simulink model "EKF_MODEL_needfix"  (R2023b)
settings: Solver=ode23tb  StartTime=0.0  StopTime=30  FixedStep=.001  RelTol=2e-1  EnableMultiTasking=on
StartFcn:
  | %tic
StopFcn:
  | %toc
model workspace (MAT data in the model file):
  DLCXref = [0 6.1 6.2 18 33 33.5 45 50 60]
  DLCXrefStanley = [0 1.2 2.4 3.6 4.8 6 7.2 8.4 9.44987166868 10.0991210544 10.1 10.1008789456 ... (38 elements, 1x38)]
  DLCYref = [0 0 -5 -3.875 -3.5 1 0 0 0]
  DLCYrefStanley = [0.1375 0.1375 0.1375 0.1375 0.1375 0.1375 0.1375 0.1375 -0.203439148031 -1.09615705337 -2.2 -3.30384294663 ... (38 elements, 1x38)]
  Downshift_Speeds = [9.5625 12.9375 16.3125 19.6875 23.0625 26.4375 29.8125 33.1875 36.5625 39.9375 43.3125 46.6875 ... (28 elements, 4x7)]
  EngRevLim = 7000
  Pedal_Positions = [0.1 0.4 0.5 0.9]
  Ts = 0.01
  Upshift_Speeds = [12.9375 16.3125 19.6875 33 26.4375 29.8125 33.1875 52.5 39.9375 43.3125 46.6875 77.25 ... (28 elements, 4x7)]
  VEH : object (value not decoded)
  a = 1.515
  b = 1.504
  for_ekf : mamfis (value not decoded)
  rayDirections = [0 0 0 0 0 0 0 0 0 0 0 0 ... (363 elements, 121x3)]
  rayLengths = [20 20 20 20 20 20 20 20 20 20 20 20 ... (121 elements, 121x1)]
  rayOrigins = [0.5 0.4 0.3 0.2 0.1 0 -0.1 -0.2 -0.3 -0.4 -0.5 0.5 ... (363 elements, 121x3)]
  theta = 1
  wf = 0.75
  wr = 1.25
symbols that are objects in the model workspace (value not decoded): VEH
undefined symbols (not defined in the file): DiscIntNeverNeededParam
libraries: simulink x14, autolibutils x7, slpidlib x2, vehdynlibdriver x2, vehdynlibviscommon x2, sim3dgroundtruthsensorlib x2, autolibtranscontrolscommon x1, autolibshared x1, sharedtransform x1, sharedTrackingLibrary x1, vehdynlibscenariocommon x1, vehdynlibsens x1
(part 4 of 4)

== system EKF_MODEL_needfix/Visualization/3D Engine/3D Engine/Part Translation Concatenation ==
  BodyX : Inport
  BodyY : Inport  Port=2
  BodyZ : Inport  Port=3
  WheelFrontLeftX : Inport  Port=4
  WheelFrontRightX : Inport  Port=5
  WheelRearLeftX : Inport  Port=6
  WheelRearRightX : Inport  Port=7
  WheelFrontLeftY : Inport  Port=8
  WheelFrontRightY : Inport  Port=9
  WheelRearLeftY : Inport  Port=10
  WheelRearRightY : Inport  Port=11
  WheelFrontLeftZ : Inport  Port=12
  WheelFrontRightZ : Inport  Port=13
  WheelRearLeftZ : Inport  Port=14
  WheelRearRightZ : Inport  Port=15
  AllParts : Concatenate  NumInputs=5  Mode=Multidimensional array
  Body : Concatenate  NumInputs=3  Mode=Multidimensional array  ConcatenateDimension=2
  WheelFrontLeft : Concatenate  NumInputs=3  Mode=Multidimensional array  ConcatenateDimension=2
  WheelFrontRight : Concatenate  NumInputs=3  Mode=Multidimensional array  ConcatenateDimension=2
  WheelRearLeft : Concatenate  NumInputs=3  Mode=Multidimensional array  ConcatenateDimension=2
  WheelRearRight : Concatenate  NumInputs=3  Mode=Multidimensional array  ConcatenateDimension=2
  ConcatOut : Outport  VectorParamsAs1DForOutWhenUnconnected=off
  wires:
  BodyX/1 -> Body/1
  BodyZ/1 -> Body/3
  WheelFrontLeftX/1 -> WheelFrontLeft/1
  WheelFrontLeftZ/1 -> WheelFrontLeft/3
  WheelFrontLeftY/1 -> WheelFrontLeft/2
  BodyY/1 -> Body/2
  WheelFrontLeft/1 -> AllParts/2
  WheelRearRightX/1 -> WheelRearRight/1
  Body/1 -> AllParts/1
  WheelRearLeft/1 -> AllParts/4
  WheelFrontRight/1 -> AllParts/3
  WheelRearRightZ/1 -> WheelRearRight/3
  WheelFrontRightY/1 -> WheelFrontRight/2
  WheelFrontRightX/1 -> WheelFrontRight/1
  WheelRearRightY/1 -> WheelRearRight/2
  WheelRearLeftZ/1 -> WheelRearLeft/3
  AllParts/1 -> ConcatOut/1
  WheelRearLeftY/1 -> WheelRearLeft/2
  WheelRearRight/1 -> AllParts/5
  WheelRearLeftX/1 -> WheelRearLeft/1
  WheelFrontRightZ/1 -> WheelFrontRight/3

== system EKF_MODEL_needfix/Visualization/3D Engine/3D Engine/Scale ==
  Constant{1..12,17,32..33} (15 alike) : Constant  OutDataTypeStr=single
  PartConcatenation : Subsystem
  ScaleOut : Outport  VectorParamsAs1DForOutWhenUnconnected=off
  wires:
  Constant10/1 -> PartConcatenation/15(WheelRearRightZ)
  Constant9/1 -> PartConcatenation/14(WheelRearRightY)
  Constant11/1 -> PartConcatenation/13(WheelRearRightX)
  Constant7/1 -> PartConcatenation/12(WheelRearLeftZ)
  Constant6/1 -> PartConcatenation/11(WheelRearLeftY)
  Constant8/1 -> PartConcatenation/10(WheelRearLeftX)
  Constant4/1 -> PartConcatenation/9(WheelFrontRightZ)
  Constant3/1 -> PartConcatenation/8(WheelFrontRightY)
  Constant5/1 -> PartConcatenation/7(WheelFrontRightX)
  Constant2/1 -> PartConcatenation/6(WheelFrontLeftZ)
  Constant1/1 -> PartConcatenation/5(WheelFrontLeftY)
  Constant33/1 -> PartConcatenation/4(WheelFrontLeftX)
  Constant32/1 -> PartConcatenation/3(BodyZ)
  Constant17/1 -> PartConcatenation/2(BodyY)
  Constant12/1 -> PartConcatenation/1(BodyX)
  PartConcatenation/1(ConcatOut) -> ScaleOut/1

== system EKF_MODEL_needfix/Controllers/Brake Pressure Control/Five-State ABS and TCS/ABSCtrlForEach/For Each Subsystem ==
  e1 : Inport  Partition=on  PartitionDimension=1  PartitionWidth=1  PartitionOffset=0
  e2 : Inport  Port=2  Partition=on  PartitionDimension=1  PartitionWidth=1  PartitionOffset=0
  Pref : Inport  Port=3  Partition=on  PartitionDimension=1  PartitionWidth=1  PartitionOffset=0
  VehSpd : Inport  Port=4
  ABSForEachWheel : Stateflow chart  InitFcn=[~]=vehdynicon('vehdynblk',gcb);  TreatAsAtomicUnit=on
  For Each : ForEach  DisableCoverage=on
  Saturation2 : Saturate  UpperLimit=1  LowerLimit=0  ZeroCross=off
  Pb : Outport  ConcatenationDimension=1
  Flag : Outport  Port=2  ConcatenationDimension=1
  wires:
  e1/1 -> ABSForEachWheel/1(e1)
  e2/1 -> ABSForEachWheel/2(e2)
  VehSpd/1 -> ABSForEachWheel/4(VehSpd)
  Saturation2/1 -> Pb/1  "BrkPrsCmdCtrl"
  ABSForEachWheel/2(Flag) -> Flag/1
  ABSForEachWheel/1(PbOutput) -> Saturation2/1
  Pref/1 -> ABSForEachWheel/3(Pref)

== system EKF_MODEL_needfix/Controllers/Brake Pressure Control/Five-State ABS and TCS/TCSCtrlForEach/For Each Subsystem ==
  e1 : Inport  Partition=on  PartitionDimension=1  PartitionWidth=1  PartitionOffset=0
  Enb : Inport  Port=2
  e2 : Inport  Port=3  Partition=on  PartitionDimension=1  PartitionWidth=1  PartitionOffset=0
  AccelFdbk : Inport  Port=4  Partition=on  PartitionDimension=1  PartitionWidth=1  PartitionOffset=0
  PbFdbk : Inport  Port=5  Partition=on  PartitionDimension=1  PartitionWidth=1  PartitionOffset=0
  ABSForEachWheel : Stateflow chart  InitFcn=[~]=vehdynicon('vehdynblk',gcb);  TreatAsAtomicUnit=on
  Discrete-Time Integrator1 : DiscreteIntegrator  IntegratorMethod=Integration: Trapezoidal  ExternalReset=rising  SampleTime=-1  LimitOutput=on  UpperSaturationLimit=1  LowerSaturationLimit=0  ICPrevOutput=DiscIntNeverNeededParam  ICPrevScaledInput=DiscIntNeverNeededParam
  For Each : ForEach  DisableCoverage=on
  IsNegative : simulink/Logic and Bit Operations/Compare To Zero  relop===  OutDataTypeStr=boolean  ZeroCross=off
  Pb : Outport  ConcatenationDimension=1
  Flag : Outport  Port=2  ConcatenationDimension=1
  wires:
  e1/1 -> ABSForEachWheel/1(e1)
  e2/1 -> ABSForEachWheel/2(e2)
  Discrete-Time Integrator1/1 -> Pb/1  "BrkPrsCmdCtrl"
  ABSForEachWheel/2(Flag) -> IsNegative/1, Flag/1
  ABSForEachWheel/1(PbOutput) -> Discrete-Time Integrator1/1
  AccelFdbk/1 -> ABSForEachWheel/3(AccelFdbk)
  Enb/1 -> ABSForEachWheel/4(Enb)
  PbFdbk/1 -> ABSForEachWheel/5(Pb)
  IsNegative/1 -> Discrete-Time Integrator1/2

== system EKF_MODEL_needfix/Controllers/Brake Pressure Control/Five-State ABS and TCS/Wheel Accel and Slip Estimator/Kappa ==
  xdot : Inport
  Omega : Inport  Port=2  PortDimensions=1  Partition=on  PartitionDimension=1  PartitionWidth=1  PartitionOffset=0
  For Each : ForEach  DisableCoverage=on
  MATLAB Function : MATLAB Function  TreatAsAtomicUnit=on
  KappaEst : Outport  ConcatenationDimension=1
  wires:
  MATLAB Function/1(KappaEst) -> KappaEst/1
  xdot/1 -> MATLAB Function/2(xdot)
  Omega/1 -> MATLAB Function/1(Omega)

== system EKF_MODEL_needfix/Controllers/Brake Pressure Control/Five-State ABS and TCS/Wheel Accel and Slip Estimator/Wheel Accel ==
  Omega : Inport  PortDimensions=1  Partition=on  PartitionDimension=1  PartitionWidth=1  PartitionOffset=0
  For Each : ForEach  DisableCoverage=on
  SG Diff : autolibutils/SG Diff  N=2  F=500  div0Tol=.001  aMode=2
  Terminator : Terminator
  WhlAccel : Outport  ConcatenationDimension=1
  wires:
  Omega/1 -> SG Diff/1
  SG Diff/1 -> Terminator/1
  SG Diff/2 -> WhlAccel/1

== system EKF_MODEL_needfix/Controllers/Transmission Controller/Transmission Controller/TCM/Neutral Select ==
  AccCmd : Inport
  EngSpd : Inport  Port=2
  Constant : Constant  Value=1200
  Constant1 : Constant  Value=1e-2
  Constant2 : Constant  Value=500
  Logical Operator : Logic  AllPortsSameDT=off  OutDataTypeStr=boolean
  Logical Operator1 : Logic  Operator=OR  AllPortsSameDT=off  OutDataTypeStr=boolean
  Relational Operator : RelationalOperator  Operator=<=  OutDataTypeStr=boolean  ZeroCross=off  RndMeth=Simplest  InputSameDT=off
  Relational Operator1 : RelationalOperator  Operator=<=  OutDataTypeStr=boolean  ZeroCross=off  RndMeth=Simplest  InputSameDT=off
  Relational Operator2 : RelationalOperator  Operator=<=  OutDataTypeStr=boolean  ZeroCross=off  RndMeth=Simplest  InputSameDT=off
  Neutral Select : Outport  VectorParamsAs1DForOutWhenUnconnected=off
  wires:
  EngSpd/1 -> Relational Operator/1, Relational Operator2/1
  Relational Operator1/1 -> Logical Operator/1
  AccCmd/1 -> Relational Operator1/1
  Constant1/1 -> Relational Operator1/2
  Logical Operator1/1 -> Neutral Select/1
  Constant/1 -> Relational Operator/2
  Relational Operator/1 -> Logical Operator/2
  Logical Operator/1 -> Logical Operator1/1
  Constant2/1 -> Relational Operator2/2
  Relational Operator2/1 -> Logical Operator1/2

== system EKF_MODEL_needfix/Controllers/Transmission Controller/Transmission Controller/TCM/TCM Shift Controller/calc ==
  note: Determine if next gear will be
      | higher or lower than current gear
  gear : Inport  OutDataTypeStr=double  PortDimensions=1
  pedal : Inport  Port=2  OutDataTypeStr=double  PortDimensions=1
  speed : Inport  Port=3  OutDataTypeStr=double  PortDimensions=1
  f : TriggerPort  TriggerType=function-call  VariantControl=Variant  StatesWhenEnabling=reset
      settings: CopyFcn=Stateflow.SLINSF.SimulinkMan.removeBlockPreDeleteFcn  PreDeleteFcn=Stateflow.SLINSF.SimulinkMan.unsafePredeleteFcn
  Add1 : Sum  Inputs=+-
  Add3 : Sum  Inputs=+-
  Add4 : Sum  Inputs=+-
  Calculate Upshift Threshold : Lookup_n-D  BreakpointsForDimension1=Pedal_Positions  BreakpointsForDimension2=1:7  Table=Upshift_Speeds  ExtrapMethod=Clip  UseLastTableValue=on  InternalRulePriority=Speed  RndMeth=Simplest
      settings: InputPortMap=u0,u1
  Calculate Downshift Threshold : Lookup_n-D  BreakpointsForDimension1=Pedal_Positions  BreakpointsForDimension2=2:8  Table=Downshift_Speeds  ExtrapMethod=Clip  UseLastTableValue=on  InternalRulePriority=Speed  RndMeth=Simplest
      settings: InputPortMap=u0,u1
  SpdThr : Outport  VectorParamsAs1DForOutWhenUnconnected=off
  wires:
  pedal/1 -> Calculate Downshift Threshold/1, Calculate Upshift Threshold/1
  gear/1 -> Calculate Downshift Threshold/2, Calculate Upshift Threshold/2
  Calculate Downshift Threshold/1 -> Add3/2
  Calculate Upshift Threshold/1 -> Add1/1
  speed/1 -> Add1/2, Add3/1
  Add1/1 -> Add4/1
  Add3/1 -> Add4/2
  Add4/1 -> SpdThr/1

== system EKF_MODEL_needfix/Controllers/Transmission Controller/Transmission Controller/TCM/TCM Shift Controller/calc_down ==
  gear : Inport  OutDataTypeStr=double  PortDimensions=1
  pedal : Inport  Port=2  OutDataTypeStr=double  PortDimensions=1
  f : TriggerPort  TriggerType=function-call  VariantControl=Variant  StatesWhenEnabling=reset
      settings: CopyFcn=Stateflow.SLINSF.SimulinkMan.removeBlockPreDeleteFcn  PreDeleteFcn=Stateflow.SLINSF.SimulinkMan.unsafePredeleteFcn
  Calculate Downshift Threshold : Lookup_n-D  BreakpointsForDimension1=Pedal_Positions  BreakpointsForDimension2=2:8  Table=Downshift_Speeds  ExtrapMethod=Clip  UseLastTableValue=on  InternalRulePriority=Speed  RndMeth=Simplest
      settings: InputPortMap=u0,u1
  down_th : Outport  VectorParamsAs1DForOutWhenUnconnected=off
  wires:
  Calculate Downshift Threshold/1 -> down_th/1
  gear/1 -> Calculate Downshift Threshold/2
  pedal/1 -> Calculate Downshift Threshold/1

== system EKF_MODEL_needfix/Controllers/Transmission Controller/Transmission Controller/TCM/TCM Shift Controller/calc_up ==
  gear : Inport  OutDataTypeStr=double  PortDimensions=1
  pedal : Inport  Port=2  OutDataTypeStr=double  PortDimensions=1
  f : TriggerPort  TriggerType=function-call  VariantControl=Variant  StatesWhenEnabling=reset
      settings: CopyFcn=Stateflow.SLINSF.SimulinkMan.removeBlockPreDeleteFcn  PreDeleteFcn=Stateflow.SLINSF.SimulinkMan.unsafePredeleteFcn
  Calculate Upshift Threshold : Lookup_n-D  BreakpointsForDimension1=Pedal_Positions  BreakpointsForDimension2=1:7  Table=Upshift_Speeds  ExtrapMethod=Clip  UseLastTableValue=on  InternalRulePriority=Speed  RndMeth=Simplest
      settings: InputPortMap=u0,u1
  up_th : Outport  VectorParamsAs1DForOutWhenUnconnected=off
  wires:
  Calculate Upshift Threshold/1 -> up_th/1
  pedal/1 -> Calculate Upshift Threshold/1
  gear/1 -> Calculate Upshift Threshold/2

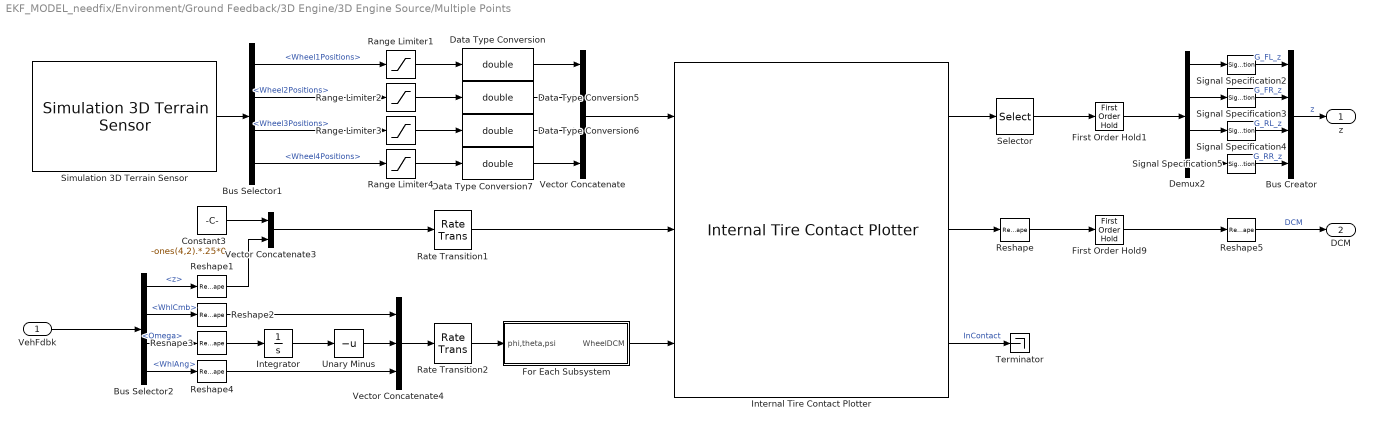
== system EKF_MODEL_needfix/Environment/Ground Feedback/3D Engine/3D Engine Source/Multiple Points ==
  VehFdbk : Inport
  Bus Creator : BusCreator  Inputs=4
  Bus Selector1 : BusSelector  OutputSignals=Wheel1Positions,Wheel2Positions,Wheel3Positions,Wheel4Positions
  Bus Selector2 : BusSelector  OutputSignals=Wheels.TireFrame.z,Wheels.Steering.WhlCmb,Wheels.TireFrame.Omega,Wheels.Steering.WhlAng
  Constant3 : Constant  Value=-ones(4,2).*.25*0
  Data Type Conversion{,5..7} (4 alike) : DataTypeConversion  OutDataTypeStr=double  SaturateOnIntegerOverflow=off  RndMeth=Floor
  Demux2 : Demux
  First Order Hold1 : FirstOrderHold  OutputAlgorithm=Fast (Minimize Error)  ErrorTolerance=.001
  First Order Hold9 : FirstOrderHold  InitialOutput=reshape(repmat(eye(3),1,1,4),[],1)  OutputAlgorithm=Fast (Minimize Error)  ErrorTolerance=.001
  For Each Subsystem : Subsystem  TreatAsAtomicUnit=on
  Integrator : Integrator  WrapState=on  ZeroCross=off
  Internal Tire Contact Plotter : vehdynlibviscommon/Internal Tire Contact Plotter  dispFig=on  numAxles=2  numWheelsPerAxle=2  wheelRad=.33  wheelWidth=.235  rayOrigins=rayOrigins
  Range Limiter{1..4} (4 alike) : Saturate  UpperLimit=1e3  LowerLimit=-1e3  ZeroCross=off
  Rate Transition1 : RateTransition  Integrity=off  Deterministic=off  OutPortSampleTime=.005
  Rate Transition2 : RateTransition  Integrity=off  Deterministic=off  OutPortSampleTime=.005
  Reshape : Reshape  OutputDimensionality=Column vector (2-D)
  Reshape1 : Reshape  OutputDimensionality=Column vector (2-D)
  Reshape2 : Reshape  OutputDimensionality=Row vector (2-D)
  Reshape3 : Reshape  OutputDimensionality=Row vector (2-D)
  Reshape4 : Reshape  OutputDimensionality=Row vector (2-D)
  Reshape5 : Reshape  OutputDimensionality=Customize  OutputDimensions=[3,3,4]
  Selector : Selector  NumberOfDimensions=2  InputPortWidth=3  IndexOptions=Select all,Index vector (dialog)  Indices=[1 3],3  OutputSizes=1,1
  Signal Specification{2..5} (4 alike) : SignalSpecification  Unit=m
  Simulation 3D Terrain Sensor : sim3dgroundtruthsensorlib/Simulation 3D Terrain Sensor  Priority=1  VehicleIdentifier=SimulinkVehicle1  vehTagList={'Scene Origin'}  sensorTag=Sim3dSensor1  sensorId=1  sensorName=Sim3dSensor1  vehTag=Scene Origin  tmountOffset=[0, 0, 0]  rmountOffset=[0,0,0,]  RayOrigins=rayOrigins  RayDirections=rayDirections  RayLengths=rayLengths  NumberOfWheels=4  VisualizeTraceLines=off  SampleTime=-1  aMode=2  ID=1
  Terminator : Terminator
  Unary Minus : UnaryMinus
  Vector Concatenate : Concatenate  NumInputs=4  Mode=Multidimensional array  ConcatenateDimension=3
  Vector Concatenate3 : Concatenate  Mode=Multidimensional array  ConcatenateDimension=2
  Vector Concatenate4 : Concatenate  NumInputs=3  Mode=Multidimensional array
  z : Outport
  DCM : Outport  Port=2
  wires:
  Data Type Conversion6/1 -> Vector Concatenate/3
  Range Limiter2/1 -> Data Type Conversion5/1
  Selector/1 -> First Order Hold1/1
  Signal Specification5/1 -> Bus Creator/4  "G_RR_z"
  Bus Selector1/3 -> Range Limiter3/1  "<Wheel3Positions>"
  Demux2/2 -> Signal Specification3/1
  Range Limiter3/1 -> Data Type Conversion6/1
  Data Type Conversion/1 -> Vector Concatenate/1
  Data Type Conversion5/1 -> Vector Concatenate/2
  Demux2/3 -> Signal Specification4/1
  Internal Tire Contact Plotter/1 -> Selector/1
  Internal Tire Contact Plotter/3 -> Terminator/1  "InContact"
  Vector Concatenate/1 -> Internal Tire Contact Plotter/1
  Data Type Conversion7/1 -> Vector Concatenate/4
  Bus Selector1/1 -> Range Limiter1/1  "<Wheel1Positions>"
  Range Limiter4/1 -> Data Type Conversion7/1
  Demux2/4 -> Signal Specification5/1
  Bus Creator/1 -> z/1  "z"
  Signal Specification2/1 -> Bus Creator/1  "G_FL_z"
  Bus Selector1/4 -> Range Limiter4/1  "<Wheel4Positions>"
  Signal Specification3/1 -> Bus Creator/2  "G_FR_z"
  Signal Specification4/1 -> Bus Creator/3  "G_RL_z"
  Bus Selector1/2 -> Range Limiter2/1  "<Wheel2Positions>"
  Demux2/1 -> Signal Specification2/1
  Simulation 3D Terrain Sensor/1 -> Bus Selector1/1
  Range Limiter1/1 -> Data Type Conversion/1
  Reshape5/1 -> DCM/1  "DCM"
  Internal Tire Contact Plotter/2 -> Reshape/1
  Bus Selector2/3 -> Reshape3/1  "<Omega>"
  Integrator/1 -> Unary Minus/1
  Bus Selector2/2 -> Reshape2/1  "<WhlCmb>"
  Vector Concatenate3/1 -> Rate Transition1/1
  For Each Subsystem/1(WheelDCM) -> Internal Tire Contact Plotter/3
  Reshape3/1 -> Integrator/1
  Vector Concatenate4/1 -> Rate Transition2/1
  Reshape4/1 -> Vector Concatenate4/3
  Rate Transition2/1 -> For Each Subsystem/1(phi,theta,psi)
  Reshape1/1 -> Vector Concatenate3/2
  VehFdbk/1 -> Bus Selector2/1
  Bus Selector2/1 -> Reshape1/1  "<z>"
  Bus Selector2/4 -> Reshape4/1  "<WhlAng>"
  Constant3/1 -> Vector Concatenate3/1
  Reshape2/1 -> Vector Concatenate4/1
  Unary Minus/1 -> Vector Concatenate4/2
  Rate Transition1/1 -> Internal Tire Contact Plotter/2
  First Order Hold9/1 -> Reshape5/1
  Reshape/1 -> First Order Hold9/1
  First Order Hold1/1 -> Demux2/1

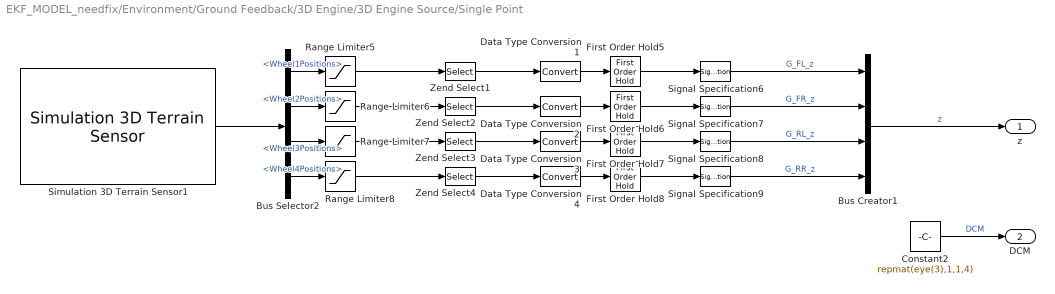
== system EKF_MODEL_needfix/Environment/Ground Feedback/3D Engine/3D Engine Source/Single Point ==
  Bus Creator1 : BusCreator  Inputs=4
  Bus Selector2 : BusSelector  OutputSignals=Wheel1Positions,Wheel2Positions,Wheel3Positions,Wheel4Positions
  Constant2 : Constant  Value=repmat(eye(3),1,1,4)  SampleTime=-1
  Data Type Conversion{1..4} (4 alike) : DataTypeConversion  SaturateOnIntegerOverflow=off  RndMeth=Floor
  First Order Hold{5..8} (4 alike) : FirstOrderHold  ErrorTolerance=1
  Range Limiter{5..8} (4 alike) : Saturate  UpperLimit=1e3  LowerLimit=-1e3  ZeroCross=off
  Signal Specification{6..9} (4 alike) : SignalSpecification  Unit=m
  Simulation 3D Terrain Sensor1 : sim3dgroundtruthsensorlib/Simulation 3D Terrain Sensor  Priority=1  vehTagList={'Scene Origin';'SimulinkVehicle1'}  sensorTag=Sim3dSensor1  sensorId=1  sensorName=Sim3dSensor1  vehTag=SimulinkVehicle1  tmountOffset=[0, 0, 0]  rmountOffset=[0,0,0,]  RayOrigins=[0 0 1]  RayDirections=[0 0 -1]  RayLengths=20  NumberOfWheels=4  VisualizeTraceLines=off  SampleTime=-1  aMode=2  ID=1
  Zend Select{1..4} (4 alike) : Selector  NumberOfDimensions=2  InputPortWidth=3  IndexOptions=Select all,Index vector (dialog)  Indices=[1 3],3  OutputSizes=1,1
  z : Outport
  DCM : Outport  Port=2
  wires:
  Signal Specification6/1 -> Bus Creator1/1  "G_FL_z"
  Simulation 3D Terrain Sensor1/1 -> Bus Selector2/1
  Bus Selector2/4 -> Range Limiter8/1  "<Wheel4Positions>"
  Zend Select1/1 -> Data Type Conversion1/1
  Signal Specification7/1 -> Bus Creator1/2  "G_FR_z"
  Bus Selector2/2 -> Range Limiter6/1  "<Wheel2Positions>"
  Data Type Conversion3/1 -> First Order Hold7/1
  Data Type Conversion4/1 -> First Order Hold8/1
  Zend Select3/1 -> Data Type Conversion3/1
  First Order Hold6/1 -> Signal Specification7/1
  Zend Select2/1 -> Data Type Conversion2/1
  Data Type Conversion2/1 -> First Order Hold6/1
  Range Limiter6/1 -> Zend Select2/1
  Data Type Conversion1/1 -> First Order Hold5/1
  First Order Hold7/1 -> Signal Specification8/1
  Zend Select4/1 -> Data Type Conversion4/1
  Range Limiter8/1 -> Zend Select4/1
  Bus Selector2/1 -> Range Limiter5/1  "<Wheel1Positions>"
  First Order Hold8/1 -> Signal Specification9/1
  Bus Selector2/3 -> Range Limiter7/1  "<Wheel3Positions>"
  Range Limiter7/1 -> Zend Select3/1
  First Order Hold5/1 -> Signal Specification6/1
  Range Limiter5/1 -> Zend Select1/1
  Signal Specification8/1 -> Bus Creator1/3  "G_RL_z"
  Signal Specification9/1 -> Bus Creator1/4  "G_RR_z"
  Bus Creator1/1 -> z/1  "z"
  Constant2/1 -> DCM/1  "DCM"

== system EKF_MODEL_needfix/Visualization/3D Engine/3D Engine/Scale/PartConcatenation ==
  BodyX : Inport
  BodyY : Inport  Port=2
  BodyZ : Inport  Port=3
  WheelFrontLeftX : Inport  Port=4
  WheelFrontLeftY : Inport  Port=5
  WheelFrontLeftZ : Inport  Port=6
  WheelFrontRightX : Inport  Port=7
  WheelFrontRightY : Inport  Port=8
  WheelFrontRightZ : Inport  Port=9
  WheelRearLeftX : Inport  Port=10
  WheelRearLeftY : Inport  Port=11
  WheelRearLeftZ : Inport  Port=12
  WheelRearRightX : Inport  Port=13
  WheelRearRightY : Inport  Port=14
  WheelRearRightZ : Inport  Port=15
  AllParts : Concatenate  NumInputs=5  Mode=Multidimensional array
  Body : Concatenate  NumInputs=3  Mode=Multidimensional array  ConcatenateDimension=2
  WheelFrontLeft : Concatenate  NumInputs=3  Mode=Multidimensional array  ConcatenateDimension=2
  WheelFrontRight : Concatenate  NumInputs=3  Mode=Multidimensional array  ConcatenateDimension=2
  WheelRearLeft : Concatenate  NumInputs=3  Mode=Multidimensional array  ConcatenateDimension=2
  WheelRearRight : Concatenate  NumInputs=3  Mode=Multidimensional array  ConcatenateDimension=2
  ConcatOut : Outport  VectorParamsAs1DForOutWhenUnconnected=off
  wires:
  BodyX/1 -> Body/1
  BodyZ/1 -> Body/3
  WheelFrontLeftX/1 -> WheelFrontLeft/1
  WheelFrontLeftZ/1 -> WheelFrontLeft/3
  WheelFrontLeftY/1 -> WheelFrontLeft/2
  BodyY/1 -> Body/2
  WheelFrontLeft/1 -> AllParts/2
  WheelRearRightX/1 -> WheelRearRight/1
  Body/1 -> AllParts/1
  WheelRearLeft/1 -> AllParts/4
  WheelFrontRight/1 -> AllParts/3
  WheelRearRightZ/1 -> WheelRearRight/3
  WheelFrontRightY/1 -> WheelFrontRight/2
  WheelFrontRightX/1 -> WheelFrontRight/1
  WheelRearRightY/1 -> WheelRearRight/2
  WheelRearLeftZ/1 -> WheelRearLeft/3
  AllParts/1 -> ConcatOut/1
  WheelRearLeftY/1 -> WheelRearLeft/2
  WheelRearRight/1 -> AllParts/5
  WheelRearLeftX/1 -> WheelRearLeft/1
  WheelFrontRightZ/1 -> WheelFrontRight/3

== system EKF_MODEL_needfix/Environment/Ground Feedback/3D Engine/3D Engine Source/Multiple Points/For Each Subsystem ==
  phi,theta,psi : Inport  Partition=on  PartitionDimension=2  PartitionWidth=1  PartitionOffset=0
  For Each : ForEach  DisableCoverage=on
  Rotation Angles to Direction Cosine Matrix1 : sharedtransform/Rotation Angles to Direction Cosine Matrix  rotationOrder=YXZ  aMode=2
  Selector5 : Selector  InputPortWidth=3  IndexOptions=Index vector (dialog)  Indices=[2 1 3]  OutputSizes=1
  WheelDCM : Outport  ConcatenationDimension=3
  wires:
  Selector5/1 -> Rotation Angles to Direction Cosine Matrix1/1
  Rotation Angles to Direction Cosine Matrix1/1 -> WheelDCM/1
  phi,theta,psi/1 -> Selector5/1

== stateflow chart EKF_MODEL_needfix/Controllers/Transmission Controller/Transmission Controller/TCM/TCM Shift Controller ==
  settings: sampleTime=0.01
  state GearCmd [parallel]
    settings: executionOrder=1
    state Neutral
      en:
      GearCmd = 0;
    state G1
      en:
      GearCmd = 1;
    state G2
      en:
      GearCmd = 2;
      du:
      [SpdThr] = calc(2,pedal,speed);
    state G3
      en:
      GearCmd = 3;
      du:
      [SpdThr] = calc(3,pedal,speed);
    state G8
      en:
      GearCmd = 8;
    state G7
      en:
      GearCmd = 7;
    state G6
      en:
      GearCmd = 6;
    state G5
      en:GearCmd=5;
      du:[SpdThr]=calc(5,pedal,speed);
    state G4
      en:
      GearCmd = 4;
      du:
      [SpdThr] = calc(4,pedal,speed);
    (default) -> Neutral
    Neutral -> G1 : [~Neutral]
    G1 -> G2 [order 1] : Up
    G2 -> G3 [order 1] : Up
    G1 -> Neutral [order 2] : [Neutral]
    G2 -> G1 [order 2] : Down
    G3 -> G2 [order 2] : Down
    G3 -> G4 [order 1] : Up
    G4 -> G3 [order 2] : Down
    G7 -> G8 [order 1] : Up
    G5 -> G6 [order 1] : Up
    G6 -> G7 [order 1] : Up
    G4 -> G5 [order 1] : Up
    G5 -> G4 [order 2] : Down
    G6 -> G5 [order 2] : Down
    G7 -> G6 [order 2] : Down
    G8 -> G7 : Down
  state SelectionState [parallel]
    du:[up_th]=calc_up(GearCmd,pedal);
    du:[down_th]=calc_down(GearCmd,pedal);
    settings: executionOrder=2
    state SteadyState
      en:
      clutchControl = 0;
    state preDownShifting
    state preUpShifting
    state UpShifting
      en:
      GearCmd = GearCmd + 0.5;
    state DownShifting
      en:
      GearCmd = GearCmd - 0.5;
    (default) -> SteadyState
    SteadyState -> (junction 62) [order 1] : [speed < down_th && ...
        | GearCmd >1]
    SteadyState -> (junction 128) [order 2] : [speed > up_th &&...
        | GearCmd <= 5 && ...
        | floor(GearCmd) == GearCmd]
    (junction 62) -> preDownShifting
    (junction 128) -> preUpShifting
    (junction 168) -> SteadyState
    (junction 23) -> SteadyState
    (junction 161) -> SteadyState
    preDownShifting -> (junction 168) [order 2] : [speed >= down_th]
    preUpShifting -> (junction 161) [order 2] : [speed <= up_th]
    preUpShifting -> UpShifting [order 1] : after(0.5,sec)
        | [speed>up_th]
    preDownShifting -> DownShifting [order 1] : after(0.5, sec)
        | [speed < down_th - 2]
    DownShifting -> (junction 23) : {GearCmd.Down;}
    UpShifting -> (junction 23) : {GearCmd.Up;}
  state up_th = calc_up(gear,pedal) [function]
  state down_th = calc_down(gear,pedal) [function]
  state SpdThr = calc(gear,pedal,speed) [function]
  data: gear function_input double size=1; pedal function_input double size=1; up_th function_output; gear function_input double size=1; pedal function_input double size=1; down_th function_output; gear function_input double size=1; pedal function_input double size=1; SpdThr function_output; speed function_input double size=1; GearCmd output int8; speed input; pedal input; clutchControl local double; SpdThr local double; Neutral input; up_th local double; down_th local double
  events: Up local EITHER_EDGE_EVENT; Down local EITHER_EDGE_EVENT

== stateflow chart EKF_MODEL_needfix/Controllers/Brake Pressure Control/Five-State ABS and TCS/TCSCtrlForEach/For Each Subsystem/ABSForEachWheel ==
  state TCSOff
    entry:
    PbOutput = 0;
    Flag = 0;
    during:
    PbOutput = 0;
  state TCSRelease
    entry:
    PbOutput = v4;
  state Normal
    entry:
    PbOutput = 0;
    Flag = 0;
    during:
    PbOutput = 0;
  state TCSOn
    state Phase1
      entry:
      PbOutput = v1;
      Flag = 1;
    state Phase5
      entry:
      PbOutput = v5;
      Flag = 5;
    state Phase2
      entry:
      PbOutput = 0;
      Flag = 2;
    state Phase4
      entry:
      PbOutput = 0;
      Flag = 4;
    state Phase3
      entry:
      PbOutput = v4;
      Flag = 3;
    (default) -> Phase1
    Phase5 -> Phase1 : [e2 > a2]
    Phase1 -> Phase2 : [e2 <= b]
    Phase4 -> Phase5 : [e2 >= a1]
    Phase2 -> Phase3 : [e2 <= A]
    Phase3 -> Phase4 : [e2 > A]
  (default) -> TCSOff
  TCSRelease -> TCSOff : [Pb <= 0 || AccelFdbk <= 0.2]
  Normal -> TCSOff [order 2] : [AccelFdbk <= 0]
  TCSOn -> TCSRelease : [ AccelFdbk <= 0.2]
  TCSOff -> Normal : [AccelFdbk > 0 && e2 > a2 && Enb > 0.3]
  Normal -> TCSOn [order 1] : [e1 > 0]
  data: e1 input; e2 input; PbOutput output; Flag output; b parameter; v1 parameter; v4 parameter; v5 parameter; A parameter; a2 parameter; a1 parameter; AccelFdbk input; Enb input; Pb input

== matlab function EKF_MODEL_needfix/Simulink Function/MATLAB Function ==
  data: x1 input; y output; x2 input; x3 input
function y = fcn(x1,x2,x3)

y = x1+0.01*x2*x3;

== matlab function EKF_MODEL_needfix/Subsystem1/MATLAB Function ==
  settings: updateMethod=DISCRETE
  data: variance input; randomMatrix output
function randomMatrix = generateGaussianRandomMatrix(variance)
    % 生成具有高斯分布的4x1矩阵
    % 输入参数：
    %   variance: 方差
    % 输出参数：
    %   randomMatrix: 4x1矩阵

    % 使用 randn 函数生成高斯分布的随机值，并构建4x1矩阵
    randomValues = sqrt(variance) * randn(4, 1);

    % 将随机值存储为4x1矩阵
    randomMatrix = randomValues;
end

== matlab function EKF_MODEL_needfix/imu signal/MATLAB Function1 ==
  data: variance input; randomMatrix output
function randomMatrix = generateGaussianRandomMatrix(variance)
    % 生成具有高斯分布的4x1矩阵
    % 输入参数：
    %   variance: 方差
    % 输出参数：
    %   randomMatrix: 4x1矩阵

    % 使用 randn 函数生成高斯分布的随机值，并构建4x1矩阵
    randomValues = sqrt(variance) * randn(3, 1);

    % 将随机值存储为4x1矩阵
    randomMatrix = randomValues;
end

== matlab function EKF_MODEL_needfix/Simulink Function/MATLAB Function1 ==
  data: x1 input; y output; x2 input; x3 input
function y = fcn(x1,x2,x3)

y = x2-0.01*x1*x3;

== matlab function EKF_MODEL_needfix/Simulink Function/MATLAB Function2 ==
  data: x1 input; y output; x2 input; x3 input
function y = fcn(x1,x2,x3)

y = 0;

== matlab function EKF_MODEL_needfix/Simulink Function1/MATLAB Function ==
  data: theta input; y output; wf input; wr input; a input
function y = fcn(theta,wf,wr,a)

y = [cos(theta) sin(theta) -wf/2*cos(theta)+a*sin(theta); cos(theta) sin(theta) wf/2*cos(theta)+a*sin(theta); 1 0 -wr/2; 1 0 wr/2];

== matlab function EKF_MODEL_needfix/Simulink Function2/MATLAB Function3 ==
  data: x1 input; A output; x2 input; x3 input
function A = fcn(x1,x2,x3)


Ts=0.01;
A = [1 Ts*x3 Ts*x2; -Ts*x3 1 -Ts*x1; 0 0 0];

== matlab function EKF_MODEL_needfix/Subsystem2/MATLAB Function4 ==
  data: vehicle_speed input; slip_ratio output; wheel_speed input
function slip_ratio = calculateSlipRatio(vehicle_speed, wheel_speed)
    if max(vehicle_speed,wheel_speed)<=0.01
        slip_ratio = abs(wheel_speed - vehicle_speed) / 0.01;
    else
        slip_ratio = abs(wheel_speed - vehicle_speed) / max(vehicle_speed,wheel_speed);
    end

== matlab function EKF_MODEL_needfix/Subsystem1/MATLAB Function2 ==
  data: u input; y output
function y = fcn(u)
   
y = [u 0 0 0;
     0 u 0 0;
     0 0 u 0;
     0 0 0 u];

== matlab function EKF_MODEL_needfix/Subsystem2/MATLAB Function1 ==
  data: vehicle_speed input; slip_ratio output; wheel_speed input
function slip_ratio = calculateSlipRatio(vehicle_speed, wheel_speed)
    if max(vehicle_speed,wheel_speed)<=0.01
        slip_ratio = abs(wheel_speed - vehicle_speed) / 0.01;
    else
        slip_ratio = abs(wheel_speed - vehicle_speed) / max(vehicle_speed,wheel_speed);
    end

== matlab function EKF_MODEL_needfix/Subsystem2/MATLAB Function2 ==
  data: vehicle_speed input; slip_ratio output; wheel_speed input
function slip_ratio = calculateSlipRatio(vehicle_speed, wheel_speed)
    if max(vehicle_speed,wheel_speed)<=0.01
        slip_ratio = abs(wheel_speed - vehicle_speed) / 0.01;
    else
        slip_ratio = abs(wheel_speed - vehicle_speed) / max(vehicle_speed,wheel_speed);
    end

== matlab function EKF_MODEL_needfix/Controllers/Brake Pressure Control/Bang Bang ABS/Kappa/MATLAB Function ==
  data: Omega input; xdot input; KappaEst output
function KappaEst = fcn(Omega, xdot)

Re = 0.29;
KappaEst = 0;
WhlSpd = Omega * Re;

if xdot*WhlSpd ~= 0
    KappaEst = (WhlSpd - xdot)/max([abs(xdot) abs(WhlSpd)]);
end

== matlab function EKF_MODEL_needfix/Subsystem2/MATLAB Function3 ==
  data: vehicle_speed input; slip_ratio output; wheel_speed input
function slip_ratio = calculateSlipRatio(vehicle_speed, wheel_speed)
    if max(vehicle_speed,wheel_speed)<=0.01
        slip_ratio = abs(wheel_speed - vehicle_speed) / 0.01;
    else
        slip_ratio = abs(wheel_speed - vehicle_speed) / max(vehicle_speed,wheel_speed);
    end

== matlab function EKF_MODEL_needfix/Controllers/Brake Pressure Control/Five-State ABS and TCS/Wheel Accel and Slip Estimator/Kappa/MATLAB Function ==
  data: Omega input; xdot input; KappaEst output
function KappaEst = fcn(Omega, xdot)

Re = 0.29;
KappaEst = 0;
WhlSpd = Omega * Re;

if xdot*WhlSpd ~= 0
    KappaEst = (WhlSpd - xdot)/max([abs(xdot) abs(WhlSpd)]);
end

== stateflow chart EKF_MODEL_needfix/Controllers/Brake Pressure Control/Five-State ABS and TCS/ABSCtrlForEach/For Each Subsystem/ABSForEachWheel ==
  state ABSOff
    entry:
    PbOutput = Pref;
    Flag = 0;
    during:
    PbOutput = Pref;
  state Normal
    entry:
    PbOutput = Pref;
    Flag = 0;
    during:
    PbOutput = Pref;
  state ABSOn
    state Phase1
      entry:
      PbOutput = v1;
      Flag = 1;
    state Phase5
      entry:
      PbOutput = v5;
      Flag = 5;
    state Phase2
      entry:
      PbOutput = 0;
      Flag = 2;
    state Phase4
      entry:
      PbOutput = 0;
      Flag = 4;
    state Phase3
      entry:
      PbOutput = v4;
      Flag = 3;
    (default) -> Phase1
    Phase5 -> Phase1 : [e2 < a2]
    Phase1 -> Phase2 : [e2 >= b]
    Phase4 -> Phase5 : [e2 <= a1]
    Phase2 -> Phase3 : [e2 >= A]
    Phase3 -> Phase4 : [e2 < A]
  (default) -> ABSOff
  ABSOn -> ABSOff : [abs(VehSpd) < 0.1 || Pref <= 0]
  Normal -> ABSOff [order 2] : [Pref <= 0]
  ABSOff -> Normal : [Pref > 0 && e2 < a2]
  Normal -> ABSOn [order 1] : [e1 < 0]
  data: e1 input; e2 input; PbOutput output; Flag output; b parameter; v1 parameter; v4 parameter; v5 parameter; A parameter; a2 parameter; a1 parameter; Pref input; VehSpd input
